simulink model "VCU_CS75_9_30"  (R2014a)
settings: Solver=FixedStepDiscrete  StartTime=0.0  StopTime=25  FixedStep=0.0005  RelTol=1e-3
undefined symbols (not defined in the file or in its folder): APAStatus_2D4, ecucoder_acal, I_SW01_L, LDW, ST_comd, TX2D4
libraries: simulink x881, ec5744lib x37
(part 28 of 30)

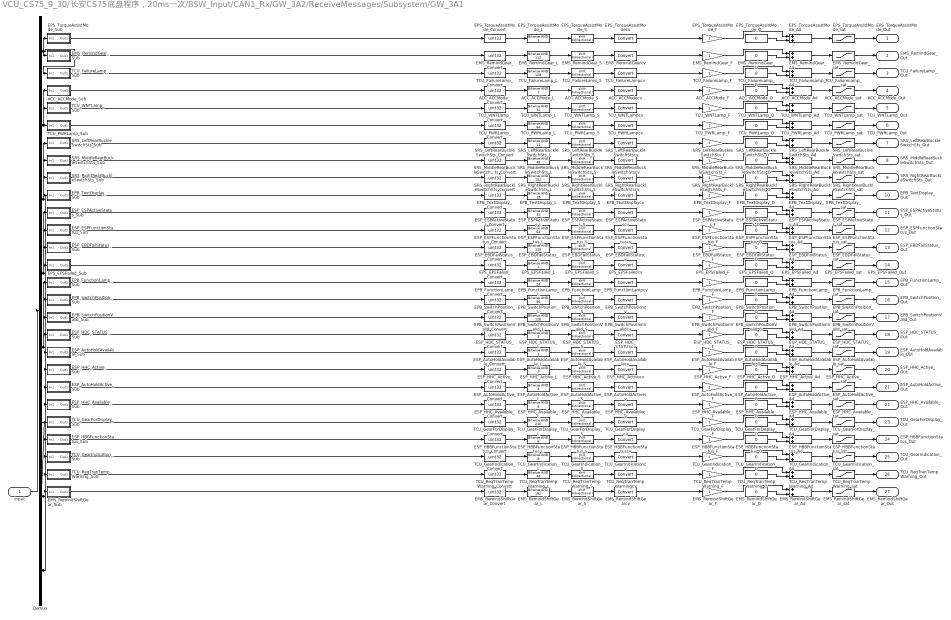
== system VCU_CS75_9_30/长安CS75底盘程序，20ms一次/BSW_Input/CAN1_Rx/GW_3A2/ReceiveMessages/Subsystem/GW_3A1 ==
  input : Inport
  ACC_ACCMode_Ad : Sum
  ACC_ACCMode_Convert : DataTypeConversion  OutDataTypeStr=uint32
  ACC_ACCMode_F : Gain
  ACC_ACCMode_L : simulink/Logic and Bit Operations/Bitwise Operator  logicop=AND  UseBitMask=on  BitMask=7  BitMaskRealWorld=Stored Integer
  ACC_ACCMode_O : Constant  Value=0  OutDataTypeStr=single
  ACC_ACCMode_S : ArithShift
  ACC_ACCMode_Sub : Subsystem
  ACC_ACCMode_sat : Saturate  UpperLimit=7  LowerLimit=0
  ACC_ACCModecv : DataTypeConversion
  Demux : Demux  Outputs=8
  EMS_RemindGear_Ad : Sum
  EMS_RemindGear_Convert : DataTypeConversion  OutDataTypeStr=uint32
  EMS_RemindGear_F : Gain
  EMS_RemindGear_L : simulink/Logic and Bit Operations/Bitwise Operator  logicop=AND  UseBitMask=on  BitMask=112  BitMaskRealWorld=Stored Integer
  EMS_RemindGear_O : Constant  Value=0  OutDataTypeStr=single
  EMS_RemindGear_S : ArithShift  BitShiftNumber=4
  EMS_RemindGear_Sub : Subsystem
  EMS_RemindGear_sat : Saturate  UpperLimit=7  LowerLimit=0
  EMS_RemindGearcv : DataTypeConversion
  EMS_RemindShiftGear_Ad : Sum
  EMS_RemindShiftGear_Convert : DataTypeConversion  OutDataTypeStr=uint32
  EMS_RemindShiftGear_F : Gain
  EMS_RemindShiftGear_L : simulink/Logic and Bit Operations/Bitwise Operator  logicop=AND  UseBitMask=on  BitMask=192  BitMaskRealWorld=Stored Integer
  EMS_RemindShiftGear_O : Constant  Value=0  OutDataTypeStr=single
  EMS_RemindShiftGear_S : ArithShift  BitShiftNumber=6
  EMS_RemindShiftGear_Sub : Subsystem
  EMS_RemindShiftGear_sat : Saturate  UpperLimit=3  LowerLimit=0
  EMS_RemindShiftGearcv : DataTypeConversion
  EPB_FunctionLamp_Ad : Sum
  EPB_FunctionLamp_Convert : DataTypeConversion  OutDataTypeStr=uint32
  EPB_FunctionLamp_F : Gain
  EPB_FunctionLamp_L : simulink/Logic and Bit Operations/Bitwise Operator  logicop=AND  UseBitMask=on  BitMask=24  BitMaskRealWorld=Stored Integer
  EPB_FunctionLamp_O : Constant  Value=0  OutDataTypeStr=single
  EPB_FunctionLamp_S : ArithShift  BitShiftNumber=3
  EPB_FunctionLamp_Sub : Subsystem
  EPB_FunctionLamp_sat : Saturate  UpperLimit=3  LowerLimit=0
  EPB_FunctionLampcv : DataTypeConversion
  EPB_SwitchPositionValid_Ad : Sum
  EPB_SwitchPositionValid_Convert : DataTypeConversion  OutDataTypeStr=uint32
  EPB_SwitchPositionValid_F : Gain
  EPB_SwitchPositionValid_L : simulink/Logic and Bit Operations/Bitwise Operator  logicop=AND  UseBitMask=on  BitMask=128  BitMaskRealWorld=Stored Integer
  EPB_SwitchPositionValid_O : Constant  Value=0  OutDataTypeStr=single
  EPB_SwitchPositionValid_S : ArithShift  BitShiftNumber=7
  EPB_SwitchPositionValid_Sub : Subsystem
  EPB_SwitchPositionValid_sat : Saturate  UpperLimit=1  LowerLimit=0
  EPB_SwitchPositionValidcv : DataTypeConversion
  EPB_SwitchPosition_Ad : Sum
  EPB_SwitchPosition_Convert : DataTypeConversion  OutDataTypeStr=uint32
  EPB_SwitchPosition_F : Gain
  EPB_SwitchPosition_L : simulink/Logic and Bit Operations/Bitwise Operator  logicop=AND  UseBitMask=on  BitMask=96  BitMaskRealWorld=Stored Integer
  EPB_SwitchPosition_O : Constant  Value=0  OutDataTypeStr=single
  EPB_SwitchPosition_S : ArithShift  BitShiftNumber=5
  EPB_SwitchPosition_Sub : Subsystem
  EPB_SwitchPosition_sat : Saturate  UpperLimit=3  LowerLimit=0
  EPB_SwitchPositioncv : DataTypeConversion
  EPB_TextDisplay_Ad : Sum
  EPB_TextDisplay_Convert : DataTypeConversion  OutDataTypeStr=uint32
  EPB_TextDisplay_F : Gain
  EPB_TextDisplay_L : simulink/Logic and Bit Operations/Bitwise Operator  logicop=AND  UseBitMask=on  BitMask=15  BitMaskRealWorld=Stored Integer
  EPB_TextDisplay_O : Constant  Value=0  OutDataTypeStr=single
  EPB_TextDisplay_S : ArithShift
  EPB_TextDisplay_Sub : Subsystem
  EPB_TextDisplay_sat : Saturate  UpperLimit=15  LowerLimit=0
  EPB_TextDisplaycv : DataTypeConversion
  EPS_EPSFailed_Ad : Sum
  EPS_EPSFailed_Convert : DataTypeConversion  OutDataTypeStr=uint32
  EPS_EPSFailed_F : Gain
  EPS_EPSFailed_L : simulink/Logic and Bit Operations/Bitwise Operator  logicop=AND  UseBitMask=on  BitMask=2  BitMaskRealWorld=Stored Integer
  EPS_EPSFailed_O : Constant  Value=0  OutDataTypeStr=single
  EPS_EPSFailed_S : ArithShift  BitShiftNumber=1
  EPS_EPSFailed_Sub : Subsystem
  EPS_EPSFailed_sat : Saturate  UpperLimit=1  LowerLimit=0
  EPS_EPSFailedcv : DataTypeConversion
  EPS_TorqueAssistMode_Ad : Sum
  EPS_TorqueAssistMode_Convert : DataTypeConversion  OutDataTypeStr=uint32
  EPS_TorqueAssistMode_F : Gain
  EPS_TorqueAssistMode_L : simulink/Logic and Bit Operations/Bitwise Operator  logicop=AND  UseBitMask=on  BitMask=3  BitMaskRealWorld=Stored Integer
  EPS_TorqueAssistMode_O : Constant  Value=0  OutDataTypeStr=single
  EPS_TorqueAssistMode_S : ArithShift
  EPS_TorqueAssistMode_Sub : Subsystem
  EPS_TorqueAssistMode_sat : Saturate  UpperLimit=3  LowerLimit=0
  EPS_TorqueAssistModecv : DataTypeConversion
  ESP_AutoHoldActive_Ad : Sum
  ESP_AutoHoldActive_Convert : DataTypeConversion  OutDataTypeStr=uint32
  ESP_AutoHoldActive_F : Gain
  ESP_AutoHoldActive_L : simulink/Logic and Bit Operations/Bitwise Operator  logicop=AND  UseBitMask=on  BitMask=4  BitMaskRealWorld=Stored Integer
  ESP_AutoHoldActive_O : Constant  Value=0  OutDataTypeStr=single
  ESP_AutoHoldActive_S : ArithShift  BitShiftNumber=2
  ESP_AutoHoldActive_Sub : Subsystem
  ESP_AutoHoldActive_sat : Saturate  UpperLimit=1  LowerLimit=0
  ESP_AutoHoldActivecv : DataTypeConversion
  ESP_AutoHoldAvailable_Ad : Sum
  ESP_AutoHoldAvailable_Convert : DataTypeConversion  OutDataTypeStr=uint32
  ESP_AutoHoldAvailable_F : Gain
  ESP_AutoHoldAvailable_L : simulink/Logic and Bit Operations/Bitwise Operator  logicop=AND  UseBitMask=on  BitMask=1  BitMaskRealWorld=Stored Integer
  ESP_AutoHoldAvailable_O : Constant  Value=0  OutDataTypeStr=single
  ESP_AutoHoldAvailable_S : ArithShift
  ESP_AutoHoldAvailable_Sub : Subsystem
  ESP_AutoHoldAvailable_sat : Saturate  UpperLimit=1  LowerLimit=0
  ESP_AutoHoldAvailablecv : DataTypeConversion
  ESP_EBDFailStatus_Ad : Sum
  ESP_EBDFailStatus_Convert : DataTypeConversion  OutDataTypeStr=uint32
  ESP_EBDFailStatus_F : Gain
  ESP_EBDFailStatus_L : simulink/Logic and Bit Operations/Bitwise Operator  logicop=AND  UseBitMask=on  BitMask=128  BitMaskRealWorld=Stored Integer
  ESP_EBDFailStatus_O : Constant  Value=0  OutDataTypeStr=single
  ESP_EBDFailStatus_S : ArithShift  BitShiftNumber=7
  ESP_EBDFailStatus_Sub : Subsystem
  ESP_EBDFailStatus_sat : Saturate  UpperLimit=1  LowerLimit=0
  ESP_EBDFailStatuscv : DataTypeConversion
  ESP_ESPActiveStatus_Ad : Sum
  ESP_ESPActiveStatus_Convert : DataTypeConversion  OutDataTypeStr=uint32
  ESP_ESPActiveStatus_F : Gain
  ESP_ESPActiveStatus_L : simulink/Logic and Bit Operations/Bitwise Operator  logicop=AND  UseBitMask=on  BitMask=32  BitMaskRealWorld=Stored Integer
  ESP_ESPActiveStatus_O : Constant  Value=0  OutDataTypeStr=single
  ESP_ESPActiveStatus_S : ArithShift  BitShiftNumber=5
  ESP_ESPActiveStatus_Sub : Subsystem
  ESP_ESPActiveStatus_sat : Saturate  UpperLimit=1  LowerLimit=0
  ESP_ESPActiveStatuscv : DataTypeConversion
  ESP_ESPFunctionStatus_Ad : Sum
  ESP_ESPFunctionStatus_Convert : DataTypeConversion  OutDataTypeStr=uint32
  ESP_ESPFunctionStatus_F : Gain
  ESP_ESPFunctionStatus_L : simulink/Logic and Bit Operations/Bitwise Operator  logicop=AND  UseBitMask=on  BitMask=64  BitMaskRealWorld=Stored Integer
  ESP_ESPFunctionStatus_O : Constant  Value=0  OutDataTypeStr=single
  ESP_ESPFunctionStatus_S : ArithShift  BitShiftNumber=6
  ESP_ESPFunctionStatus_Sub : Subsystem
  ESP_ESPFunctionStatus_sat : Saturate  UpperLimit=1  LowerLimit=0
  ESP_ESPFunctionStatuscv : DataTypeConversion
  ESP_HBBFunctionStatus_Ad : Sum
  ESP_HBBFunctionStatus_Convert : DataTypeConversion  OutDataTypeStr=uint32
  ESP_HBBFunctionStatus_F : Gain
  ESP_HBBFunctionStatus_L : simulink/Logic and Bit Operations/Bitwise Operator  logicop=AND  UseBitMask=on  BitMask=6  BitMaskRealWorld=Stored Integer
  ESP_HBBFunctionStatus_O : Constant  Value=0  OutDataTypeStr=single
  ESP_HBBFunctionStatus_S : ArithShift  BitShiftNumber=1
  ESP_HBBFunctionStatus_Sub : Subsystem
  ESP_HBBFunctionStatus_sat : Saturate  UpperLimit=3  LowerLimit=0
  ESP_HBBFunctionStatuscv : DataTypeConversion
  ESP_HDC_STATUS_Ad : Sum
  ESP_HDC_STATUS_Convert : DataTypeConversion  OutDataTypeStr=uint32
  ESP_HDC_STATUS_F : Gain
  ESP_HDC_STATUS_L : simulink/Logic and Bit Operations/Bitwise Operator  logicop=AND  UseBitMask=on  BitMask=3  BitMaskRealWorld=Stored Integer
  ESP_HDC_STATUS_O : Constant  Value=0  OutDataTypeStr=single
  ESP_HDC_STATUS_S : ArithShift
  ESP_HDC_STATUS_Sub : Subsystem
  ESP_HDC_STATUS_sat : Saturate  UpperLimit=3  LowerLimit=0
  ESP_HDC_STATUScv : DataTypeConversion
  ESP_HHC_Active_Ad : Sum
  ESP_HHC_Active_Convert : DataTypeConversion  OutDataTypeStr=uint32
  ESP_HHC_Active_F : Gain
  ESP_HHC_Active_L : simulink/Logic and Bit Operations/Bitwise Operator  logicop=AND  UseBitMask=on  BitMask=2  BitMaskRealWorld=Stored Integer
  ESP_HHC_Active_O : Constant  Value=0  OutDataTypeStr=single
  ESP_HHC_Active_S : ArithShift  BitShiftNumber=1
  ESP_HHC_Active_Sub : Subsystem
  ESP_HHC_Active_sat : Saturate  UpperLimit=1  LowerLimit=0
  ESP_HHC_Activecv : DataTypeConversion
  ESP_HHC_Available_Ad : Sum
  ESP_HHC_Available_Convert : DataTypeConversion  OutDataTypeStr=uint32
  ESP_HHC_Available_F : Gain
  ESP_HHC_Available_L : simulink/Logic and Bit Operations/Bitwise Operator  logicop=AND  UseBitMask=on  BitMask=8  BitMaskRealWorld=Stored Integer
  ESP_HHC_Available_O : Constant  Value=0  OutDataTypeStr=single
  ESP_HHC_Available_S : ArithShift  BitShiftNumber=3
  ESP_HHC_Available_Sub : Subsystem
  ESP_HHC_Available_sat : Saturate  UpperLimit=1  LowerLimit=0
  ESP_HHC_Availablecv : DataTypeConversion
  SRS_LeftRearBuckleSwitchSts_Ad : Sum
  SRS_LeftRearBuckleSwitchSts_Convert : DataTypeConversion  OutDataTypeStr=uint32
  SRS_LeftRearBuckleSwitchSts_F : Gain
  SRS_LeftRearBuckleSwitchSts_L : simulink/Logic and Bit Operations/Bitwise Operator  logicop=AND  UseBitMask=on  BitMask=12  BitMaskRealWorld=Stored Integer
  SRS_LeftRearBuckleSwitchSts_O : Constant  Value=0  OutDataTypeStr=single
  SRS_LeftRearBuckleSwitchSts_S : ArithShift  BitShiftNumber=2
  SRS_LeftRearBuckleSwitchSts_Sub : Subsystem
  SRS_LeftRearBuckleSwitchSts_sat : Saturate  UpperLimit=3  LowerLimit=0
  SRS_LeftRearBuckleSwitchStscv : DataTypeConversion
  SRS_MiddleRearBuckleSwitchSts_Ad : Sum
  SRS_MiddleRearBuckleSwitchSts_Convert : DataTypeConversion  OutDataTypeStr=uint32
  SRS_MiddleRearBuckleSwitchSts_F : Gain
  SRS_MiddleRearBuckleSwitchSts_L : simulink/Logic and Bit Operations/Bitwise Operator  logicop=AND  UseBitMask=on  BitMask=48  BitMaskRealWorld=Stored Integer
  SRS_MiddleRearBuckleSwitchSts_O : Constant  Value=0  OutDataTypeStr=single
  SRS_MiddleRearBuckleSwitchSts_S : ArithShift  BitShiftNumber=4
  SRS_MiddleRearBuckleSwitchSts_Sub : Subsystem
  SRS_MiddleRearBuckleSwitchSts_sat : Saturate  UpperLimit=3  LowerLimit=0
  SRS_MiddleRearBuckleSwitchStscv : DataTypeConversion
  SRS_RightRearBuckleSwitchSts_Ad : Sum
  SRS_RightRearBuckleSwitchSts_Convert : DataTypeConversion  OutDataTypeStr=uint32
  SRS_RightRearBuckleSwitchSts_F : Gain
  SRS_RightRearBuckleSwitchSts_L : simulink/Logic and Bit Operations/Bitwise Operator  logicop=AND  UseBitMask=on  BitMask=192  BitMaskRealWorld=Stored Integer
  SRS_RightRearBuckleSwitchSts_O : Constant  Value=0  OutDataTypeStr=single
  SRS_RightRearBuckleSwitchSts_S : ArithShift  BitShiftNumber=6
  SRS_RightRearBuckleSwitchSts_Sub : Subsystem
  SRS_RightRearBuckleSwitchSts_sat : Saturate  UpperLimit=3  LowerLimit=0
  SRS_RightRearBuckleSwitchStscv : DataTypeConversion
  TCU_FailureLamp_Ad : Sum
  TCU_FailureLamp_Convert : DataTypeConversion  OutDataTypeStr=uint32
  TCU_FailureLamp_F : Gain
  TCU_FailureLamp_L : simulink/Logic and Bit Operations/Bitwise Operator  logicop=AND  UseBitMask=on  BitMask=128  BitMaskRealWorld=Stored Integer
  TCU_FailureLamp_O : Constant  Value=0  OutDataTypeStr=single
  TCU_FailureLamp_S : ArithShift  BitShiftNumber=7
  TCU_FailureLamp_Sub : Subsystem
  TCU_FailureLamp_sat : Saturate  UpperLimit=1  LowerLimit=0
  TCU_FailureLampcv : DataTypeConversion
  TCU_GearForDisplay_Ad : Sum
  TCU_GearForDisplay_Convert : DataTypeConversion  OutDataTypeStr=uint32
  TCU_GearForDisplay_F : Gain
  TCU_GearForDisplay_L : simulink/Logic and Bit Operations/Bitwise Operator  logicop=AND  UseBitMask=on  BitMask=240  BitMaskRealWorld=Stored Integer
  TCU_GearForDisplay_O : Constant  Value=0  OutDataTypeStr=single
  TCU_GearForDisplay_S : ArithShift  BitShiftNumber=4
  TCU_GearForDisplay_Sub : Subsystem
  TCU_GearForDisplay_sat : Saturate  UpperLimit=15  LowerLimit=0
  TCU_GearForDisplaycv : DataTypeConversion
  TCU_GearIndication_Ad : Sum
  TCU_GearIndication_Convert : DataTypeConversion  OutDataTypeStr=uint32
  TCU_GearIndication_F : Gain
  TCU_GearIndication_L : simulink/Logic and Bit Operations/Bitwise Operator  logicop=AND  UseBitMask=on  BitMask=8  BitMaskRealWorld=Stored Integer
  TCU_GearIndication_O : Constant  Value=0  OutDataTypeStr=single
  TCU_GearIndication_S : ArithShift  BitShiftNumber=3
  TCU_GearIndication_Sub : Subsystem
  TCU_GearIndication_sat : Saturate  UpperLimit=1  LowerLimit=0
  TCU_GearIndicationcv : DataTypeConversion
  TCU_PWRLamp_Ad : Sum
  TCU_PWRLamp_Convert : DataTypeConversion  OutDataTypeStr=uint32
  TCU_PWRLamp_F : Gain
  TCU_PWRLamp_L : simulink/Logic and Bit Operations/Bitwise Operator  logicop=AND  UseBitMask=on  BitMask=64  BitMaskRealWorld=Stored Integer
  TCU_PWRLamp_O : Constant  Value=0  OutDataTypeStr=single
  TCU_PWRLamp_S : ArithShift  BitShiftNumber=6
  TCU_PWRLamp_Sub : Subsystem
  TCU_PWRLamp_sat : Saturate  UpperLimit=1  LowerLimit=0
  TCU_PWRLampcv : DataTypeConversion
  TCU_ReqTranTempWarning_Ad : Sum
  TCU_ReqTranTempWarning_Convert : DataTypeConversion  OutDataTypeStr=uint32
  TCU_ReqTranTempWarning_F : Gain
  TCU_ReqTranTempWarning_L : simulink/Logic and Bit Operations/Bitwise Operator  logicop=AND  UseBitMask=on  BitMask=48  BitMaskRealWorld=Stored Integer
  TCU_ReqTranTempWarning_O : Constant  Value=0  OutDataTypeStr=single
  TCU_ReqTranTempWarning_S : ArithShift  BitShiftNumber=4
  TCU_ReqTranTempWarning_Sub : Subsystem
  TCU_ReqTranTempWarning_sat : Saturate  UpperLimit=3  LowerLimit=0
  TCU_ReqTranTempWarningcv : DataTypeConversion
  TCU_WNTLamp_Ad : Sum
  TCU_WNTLamp_Convert : DataTypeConversion  OutDataTypeStr=uint32
  TCU_WNTLamp_F : Gain
  TCU_WNTLamp_L : simulink/Logic and Bit Operations/Bitwise Operator  logicop=AND  UseBitMask=on  BitMask=32  BitMaskRealWorld=Stored Integer
  TCU_WNTLamp_O : Constant  Value=0  OutDataTypeStr=single
  TCU_WNTLamp_S : ArithShift  BitShiftNumber=5
  TCU_WNTLamp_Sub : Subsystem
  TCU_WNTLamp_sat : Saturate  UpperLimit=1  LowerLimit=0
  TCU_WNTLampcv : DataTypeConversion
  EPS_TorqueAssistMode_Out : Outport
  EMS_RemindGear_Out : Outport  Port=2
  TCU_FailureLamp_Out : Outport  Port=3
  ACC_ACCMode_Out : Outport  Port=4
  TCU_WNTLamp_Out : Outport  Port=5
  TCU_PWRLamp_Out : Outport  Port=6
  SRS_LeftRearBuckleSwitchSts_Out : Outport  Port=7
  SRS_MiddleRearBuckleSwitchSts_Out : Outport  Port=8
  SRS_RightRearBuckleSwitchSts_Out : Outport  Port=9
  EPB_TextDisplay_Out : Outport  Port=10
  ESP_ESPActiveStatus_Out : Outport  Port=11
  ESP_ESPFunctionStatus_Out : Outport  Port=12
  ESP_EBDFailStatus_Out : Outport  Port=13
  EPS_EPSFailed_Out : Outport  Port=14
  EPB_FunctionLamp_Out : Outport  Port=15
  EPB_SwitchPosition_Out : Outport  Port=16
  EPB_SwitchPositionValid_Out : Outport  Port=17
  ESP_HDC_STATUS_Out : Outport  Port=18
  ESP_AutoHoldAvailable_Out : Outport  Port=19
  ESP_HHC_Active_Out : Outport  Port=20
  ESP_AutoHoldActive_Out : Outport  Port=21
  ESP_HHC_Available_Out : Outport  Port=22
  TCU_GearForDisplay_Out : Outport  Port=23
  ESP_HBBFunctionStatus_Out : Outport  Port=24
  TCU_GearIndication_Out : Outport  Port=25
  TCU_ReqTranTempWarning_Out : Outport  Port=26
  EMS_RemindShiftGear_Out : Outport  Port=27
  wires:
  input/1 -> Demux/1
  EMS_RemindShiftGearcv/1 -> EMS_RemindShiftGear_F/1
  EMS_RemindShiftGear_S/1 -> EMS_RemindShiftGearcv/1
  EMS_RemindShiftGear_L/1 -> EMS_RemindShiftGear_S/1
  EMS_RemindShiftGear_Convert/1 -> EMS_RemindShiftGear_L/1
  EMS_RemindShiftGear_Sub/1(Out1) -> EMS_RemindShiftGear_Convert/1
  EMS_RemindShiftGear_sat/1 -> EMS_RemindShiftGear_Out/1
  EMS_RemindShiftGear_Ad/1 -> EMS_RemindShiftGear_sat/1
  EMS_RemindShiftGear_O/1 -> EMS_RemindShiftGear_Ad/2
  EMS_RemindShiftGear_F/1 -> EMS_RemindShiftGear_Ad/1
  TCU_ReqTranTempWarningcv/1 -> TCU_ReqTranTempWarning_F/1
  TCU_ReqTranTempWarning_S/1 -> TCU_ReqTranTempWarningcv/1
  TCU_ReqTranTempWarning_L/1 -> TCU_ReqTranTempWarning_S/1
  TCU_ReqTranTempWarning_Convert/1 -> TCU_ReqTranTempWarning_L/1
  TCU_ReqTranTempWarning_Sub/1(Out1) -> TCU_ReqTranTempWarning_Convert/1
  TCU_ReqTranTempWarning_sat/1 -> TCU_ReqTranTempWarning_Out/1
  TCU_ReqTranTempWarning_Ad/1 -> TCU_ReqTranTempWarning_sat/1
  TCU_ReqTranTempWarning_O/1 -> TCU_ReqTranTempWarning_Ad/2
  TCU_ReqTranTempWarning_F/1 -> TCU_ReqTranTempWarning_Ad/1
  TCU_GearIndicationcv/1 -> TCU_GearIndication_F/1
  TCU_GearIndication_S/1 -> TCU_GearIndicationcv/1
  TCU_GearIndication_L/1 -> TCU_GearIndication_S/1
  TCU_GearIndication_Convert/1 -> TCU_GearIndication_L/1
  TCU_GearIndication_Sub/1(Out1) -> TCU_GearIndication_Convert/1
  TCU_GearIndication_sat/1 -> TCU_GearIndication_Out/1
  TCU_GearIndication_Ad/1 -> TCU_GearIndication_sat/1
  TCU_GearIndication_O/1 -> TCU_GearIndication_Ad/2
  TCU_GearIndication_F/1 -> TCU_GearIndication_Ad/1
  ESP_HBBFunctionStatuscv/1 -> ESP_HBBFunctionStatus_F/1
  ESP_HBBFunctionStatus_S/1 -> ESP_HBBFunctionStatuscv/1
  ESP_HBBFunctionStatus_L/1 -> ESP_HBBFunctionStatus_S/1
  ESP_HBBFunctionStatus_Convert/1 -> ESP_HBBFunctionStatus_L/1
  ESP_HBBFunctionStatus_Sub/1(Out1) -> ESP_HBBFunctionStatus_Convert/1
  Demux/8 -> EMS_RemindShiftGear_Sub/1(In1), TCU_ReqTranTempWarning_Sub/1(In1), TCU_GearIndication_Sub/1(In1), ESP_HBBFunctionStatus_Sub/1(In1)
  ESP_HBBFunctionStatus_sat/1 -> ESP_HBBFunctionStatus_Out/1
  ESP_HBBFunctionStatus_Ad/1 -> ESP_HBBFunctionStatus_sat/1
  ESP_HBBFunctionStatus_O/1 -> ESP_HBBFunctionStatus_Ad/2
  ESP_HBBFunctionStatus_F/1 -> ESP_HBBFunctionStatus_Ad/1
  TCU_GearForDisplaycv/1 -> TCU_GearForDisplay_F/1
  TCU_GearForDisplay_S/1 -> TCU_GearForDisplaycv/1
  TCU_GearForDisplay_L/1 -> TCU_GearForDisplay_S/1
  TCU_GearForDisplay_Convert/1 -> TCU_GearForDisplay_L/1
  TCU_GearForDisplay_Sub/1(Out1) -> TCU_GearForDisplay_Convert/1
  TCU_GearForDisplay_sat/1 -> TCU_GearForDisplay_Out/1
  TCU_GearForDisplay_Ad/1 -> TCU_GearForDisplay_sat/1
  TCU_GearForDisplay_O/1 -> TCU_GearForDisplay_Ad/2
  TCU_GearForDisplay_F/1 -> TCU_GearForDisplay_Ad/1
  ESP_HHC_Availablecv/1 -> ESP_HHC_Available_F/1
  ESP_HHC_Available_S/1 -> ESP_HHC_Availablecv/1
  ESP_HHC_Available_L/1 -> ESP_HHC_Available_S/1
  ESP_HHC_Available_Convert/1 -> ESP_HHC_Available_L/1
  ESP_HHC_Available_Sub/1(Out1) -> ESP_HHC_Available_Convert/1
  ESP_HHC_Available_sat/1 -> ESP_HHC_Available_Out/1
  ESP_HHC_Available_Ad/1 -> ESP_HHC_Available_sat/1
  ESP_HHC_Available_O/1 -> ESP_HHC_Available_Ad/2
  ESP_HHC_Available_F/1 -> ESP_HHC_Available_Ad/1
  ESP_AutoHoldActivecv/1 -> ESP_AutoHoldActive_F/1
  ESP_AutoHoldActive_S/1 -> ESP_AutoHoldActivecv/1
  ESP_AutoHoldActive_L/1 -> ESP_AutoHoldActive_S/1
  ESP_AutoHoldActive_Convert/1 -> ESP_AutoHoldActive_L/1
  ESP_AutoHoldActive_Sub/1(Out1) -> ESP_AutoHoldActive_Convert/1
  ESP_AutoHoldActive_sat/1 -> ESP_AutoHoldActive_Out/1
  ESP_AutoHoldActive_Ad/1 -> ESP_AutoHoldActive_sat/1
  ESP_AutoHoldActive_O/1 -> ESP_AutoHoldActive_Ad/2
  ESP_AutoHoldActive_F/1 -> ESP_AutoHoldActive_Ad/1
  ESP_HHC_Activecv/1 -> ESP_HHC_Active_F/1
  ESP_HHC_Active_S/1 -> ESP_HHC_Activecv/1
  ESP_HHC_Active_L/1 -> ESP_HHC_Active_S/1
  ESP_HHC_Active_Convert/1 -> ESP_HHC_Active_L/1
  ESP_HHC_Active_Sub/1(Out1) -> ESP_HHC_Active_Convert/1
  ESP_HHC_Active_sat/1 -> ESP_HHC_Active_Out/1
  ESP_HHC_Active_Ad/1 -> ESP_HHC_Active_sat/1
  ESP_HHC_Active_O/1 -> ESP_HHC_Active_Ad/2
  ESP_HHC_Active_F/1 -> ESP_HHC_Active_Ad/1
  ESP_AutoHoldAvailablecv/1 -> ESP_AutoHoldAvailable_F/1
  ESP_AutoHoldAvailable_S/1 -> ESP_AutoHoldAvailablecv/1
  ESP_AutoHoldAvailable_L/1 -> ESP_AutoHoldAvailable_S/1
  ESP_AutoHoldAvailable_Convert/1 -> ESP_AutoHoldAvailable_L/1
  ESP_AutoHoldAvailable_Sub/1(Out1) -> ESP_AutoHoldAvailable_Convert/1
  Demux/7 -> TCU_GearForDisplay_Sub/1(In1), ESP_HHC_Available_Sub/1(In1), ESP_AutoHoldActive_Sub/1(In1), ESP_HHC_Active_Sub/1(In1), ESP_AutoHoldAvailable_Sub/1(In1)
  ESP_AutoHoldAvailable_sat/1 -> ESP_AutoHoldAvailable_Out/1
  ESP_AutoHoldAvailable_Ad/1 -> ESP_AutoHoldAvailable_sat/1
  ESP_AutoHoldAvailable_O/1 -> ESP_AutoHoldAvailable_Ad/2
  ESP_AutoHoldAvailable_F/1 -> ESP_AutoHoldAvailable_Ad/1
  ESP_HDC_STATUScv/1 -> ESP_HDC_STATUS_F/1
  ESP_HDC_STATUS_S/1 -> ESP_HDC_STATUScv/1
  ESP_HDC_STATUS_L/1 -> ESP_HDC_STATUS_S/1
  ESP_HDC_STATUS_Convert/1 -> ESP_HDC_STATUS_L/1
  ESP_HDC_STATUS_Sub/1(Out1) -> ESP_HDC_STATUS_Convert/1
  Demux/6 -> ESP_HDC_STATUS_Sub/1(In1)
  ESP_HDC_STATUS_sat/1 -> ESP_HDC_STATUS_Out/1
  ESP_HDC_STATUS_Ad/1 -> ESP_HDC_STATUS_sat/1
  ESP_HDC_STATUS_O/1 -> ESP_HDC_STATUS_Ad/2
  ESP_HDC_STATUS_F/1 -> ESP_HDC_STATUS_Ad/1
  EPB_SwitchPositionValidcv/1 -> EPB_SwitchPositionValid_F/1
  EPB_SwitchPositionValid_S/1 -> EPB_SwitchPositionValidcv/1
  EPB_SwitchPositionValid_L/1 -> EPB_SwitchPositionValid_S/1
  EPB_SwitchPositionValid_Convert/1 -> EPB_SwitchPositionValid_L/1
  EPB_SwitchPositionValid_Sub/1(Out1) -> EPB_SwitchPositionValid_Convert/1
  EPB_SwitchPositionValid_sat/1 -> EPB_SwitchPositionValid_Out/1
  EPB_SwitchPositionValid_Ad/1 -> EPB_SwitchPositionValid_sat/1
  EPB_SwitchPositionValid_O/1 -> EPB_SwitchPositionValid_Ad/2
  EPB_SwitchPositionValid_F/1 -> EPB_SwitchPositionValid_Ad/1
  EPB_SwitchPositioncv/1 -> EPB_SwitchPosition_F/1
  EPB_SwitchPosition_S/1 -> EPB_SwitchPositioncv/1
  EPB_SwitchPosition_L/1 -> EPB_SwitchPosition_S/1
  EPB_SwitchPosition_Convert/1 -> EPB_SwitchPosition_L/1
  EPB_SwitchPosition_Sub/1(Out1) -> EPB_SwitchPosition_Convert/1
  EPB_SwitchPosition_sat/1 -> EPB_SwitchPosition_Out/1
  EPB_SwitchPosition_Ad/1 -> EPB_SwitchPosition_sat/1
  EPB_SwitchPosition_O/1 -> EPB_SwitchPosition_Ad/2
  EPB_SwitchPosition_F/1 -> EPB_SwitchPosition_Ad/1
  EPB_FunctionLampcv/1 -> EPB_FunctionLamp_F/1
  EPB_FunctionLamp_S/1 -> EPB_FunctionLampcv/1
  EPB_FunctionLamp_L/1 -> EPB_FunctionLamp_S/1
  EPB_FunctionLamp_Convert/1 -> EPB_FunctionLamp_L/1
  EPB_FunctionLamp_Sub/1(Out1) -> EPB_FunctionLamp_Convert/1
  EPB_FunctionLamp_sat/1 -> EPB_FunctionLamp_Out/1
  EPB_FunctionLamp_Ad/1 -> EPB_FunctionLamp_sat/1
  EPB_FunctionLamp_O/1 -> EPB_FunctionLamp_Ad/2
  EPB_FunctionLamp_F/1 -> EPB_FunctionLamp_Ad/1
  EPS_EPSFailedcv/1 -> EPS_EPSFailed_F/1
  EPS_EPSFailed_S/1 -> EPS_EPSFailedcv/1
  EPS_EPSFailed_L/1 -> EPS_EPSFailed_S/1
  EPS_EPSFailed_Convert/1 -> EPS_EPSFailed_L/1
  EPS_EPSFailed_Sub/1(Out1) -> EPS_EPSFailed_Convert/1
  Demux/5 -> EPB_SwitchPositionValid_Sub/1(In1), EPB_SwitchPosition_Sub/1(In1), EPB_FunctionLamp_Sub/1(In1), EPS_EPSFailed_Sub/1(In1)
  EPS_EPSFailed_sat/1 -> EPS_EPSFailed_Out/1
  EPS_EPSFailed_Ad/1 -> EPS_EPSFailed_sat/1
  EPS_EPSFailed_O/1 -> EPS_EPSFailed_Ad/2
  EPS_EPSFailed_F/1 -> EPS_EPSFailed_Ad/1
  ESP_EBDFailStatuscv/1 -> ESP_EBDFailStatus_F/1
  ESP_EBDFailStatus_S/1 -> ESP_EBDFailStatuscv/1
  ESP_EBDFailStatus_L/1 -> ESP_EBDFailStatus_S/1
  ESP_EBDFailStatus_Convert/1 -> ESP_EBDFailStatus_L/1
  ESP_EBDFailStatus_Sub/1(Out1) -> ESP_EBDFailStatus_Convert/1
  ESP_EBDFailStatus_sat/1 -> ESP_EBDFailStatus_Out/1
  ESP_EBDFailStatus_Ad/1 -> ESP_EBDFailStatus_sat/1
  ESP_EBDFailStatus_O/1 -> ESP_EBDFailStatus_Ad/2
  ESP_EBDFailStatus_F/1 -> ESP_EBDFailStatus_Ad/1
  ESP_ESPFunctionStatuscv/1 -> ESP_ESPFunctionStatus_F/1
  ESP_ESPFunctionStatus_S/1 -> ESP_ESPFunctionStatuscv/1
  ESP_ESPFunctionStatus_L/1 -> ESP_ESPFunctionStatus_S/1
  ESP_ESPFunctionStatus_Convert/1 -> ESP_ESPFunctionStatus_L/1
  ESP_ESPFunctionStatus_Sub/1(Out1) -> ESP_ESPFunctionStatus_Convert/1
  ESP_ESPFunctionStatus_sat/1 -> ESP_ESPFunctionStatus_Out/1
  ESP_ESPFunctionStatus_Ad/1 -> ESP_ESPFunctionStatus_sat/1
  ESP_ESPFunctionStatus_O/1 -> ESP_ESPFunctionStatus_Ad/2
  ESP_ESPFunctionStatus_F/1 -> ESP_ESPFunctionStatus_Ad/1
  ESP_ESPActiveStatuscv/1 -> ESP_ESPActiveStatus_F/1
  ESP_ESPActiveStatus_S/1 -> ESP_ESPActiveStatuscv/1
  ESP_ESPActiveStatus_L/1 -> ESP_ESPActiveStatus_S/1
  ESP_ESPActiveStatus_Convert/1 -> ESP_ESPActiveStatus_L/1
  ESP_ESPActiveStatus_Sub/1(Out1) -> ESP_ESPActiveStatus_Convert/1
  ESP_ESPActiveStatus_sat/1 -> ESP_ESPActiveStatus_Out/1
  ESP_ESPActiveStatus_Ad/1 -> ESP_ESPActiveStatus_sat/1
  ESP_ESPActiveStatus_O/1 -> ESP_ESPActiveStatus_Ad/2
  ESP_ESPActiveStatus_F/1 -> ESP_ESPActiveStatus_Ad/1
  EPB_TextDisplaycv/1 -> EPB_TextDisplay_F/1
  EPB_TextDisplay_S/1 -> EPB_TextDisplaycv/1
  EPB_TextDisplay_L/1 -> EPB_TextDisplay_S/1
  EPB_TextDisplay_Convert/1 -> EPB_TextDisplay_L/1
  EPB_TextDisplay_Sub/1(Out1) -> EPB_TextDisplay_Convert/1
  Demux/4 -> ESP_EBDFailStatus_Sub/1(In1), ESP_ESPFunctionStatus_Sub/1(In1), ESP_ESPActiveStatus_Sub/1(In1), EPB_TextDisplay_Sub/1(In1)
  EPB_TextDisplay_sat/1 -> EPB_TextDisplay_Out/1
  EPB_TextDisplay_Ad/1 -> EPB_TextDisplay_sat/1
  EPB_TextDisplay_O/1 -> EPB_TextDisplay_Ad/2
  EPB_TextDisplay_F/1 -> EPB_TextDisplay_Ad/1
  SRS_RightRearBuckleSwitchStscv/1 -> SRS_RightRearBuckleSwitchSts_F/1
  SRS_RightRearBuckleSwitchSts_S/1 -> SRS_RightRearBuckleSwitchStscv/1
  SRS_RightRearBuckleSwitchSts_L/1 -> SRS_RightRearBuckleSwitchSts_S/1
  SRS_RightRearBuckleSwitchSts_Convert/1 -> SRS_RightRearBuckleSwitchSts_L/1
  SRS_RightRearBuckleSwitchSts_Sub/1(Out1) -> SRS_RightRearBuckleSwitchSts_Convert/1
  SRS_RightRearBuckleSwitchSts_sat/1 -> SRS_RightRearBuckleSwitchSts_Out/1
  SRS_RightRearBuckleSwitchSts_Ad/1 -> SRS_RightRearBuckleSwitchSts_sat/1
  SRS_RightRearBuckleSwitchSts_O/1 -> SRS_RightRearBuckleSwitchSts_Ad/2
  SRS_RightRearBuckleSwitchSts_F/1 -> SRS_RightRearBuckleSwitchSts_Ad/1
  SRS_MiddleRearBuckleSwitchStscv/1 -> SRS_MiddleRearBuckleSwitchSts_F/1
  SRS_MiddleRearBuckleSwitchSts_S/1 -> SRS_MiddleRearBuckleSwitchStscv/1
  SRS_MiddleRearBuckleSwitchSts_L/1 -> SRS_MiddleRearBuckleSwitchSts_S/1
  SRS_MiddleRearBuckleSwitchSts_Convert/1 -> SRS_MiddleRearBuckleSwitchSts_L/1
  SRS_MiddleRearBuckleSwitchSts_Sub/1(Out1) -> SRS_MiddleRearBuckleSwitchSts_Convert/1
  SRS_MiddleRearBuckleSwitchSts_sat/1 -> SRS_MiddleRearBuckleSwitchSts_Out/1
  SRS_MiddleRearBuckleSwitchSts_Ad/1 -> SRS_MiddleRearBuckleSwitchSts_sat/1
  SRS_MiddleRearBuckleSwitchSts_O/1 -> SRS_MiddleRearBuckleSwitchSts_Ad/2
  SRS_MiddleRearBuckleSwitchSts_F/1 -> SRS_MiddleRearBuckleSwitchSts_Ad/1
  SRS_LeftRearBuckleSwitchStscv/1 -> SRS_LeftRearBuckleSwitchSts_F/1
  SRS_LeftRearBuckleSwitchSts_S/1 -> SRS_LeftRearBuckleSwitchStscv/1
  SRS_LeftRearBuckleSwitchSts_L/1 -> SRS_LeftRearBuckleSwitchSts_S/1
  SRS_LeftRearBuckleSwitchSts_Convert/1 -> SRS_LeftRearBuckleSwitchSts_L/1
  SRS_LeftRearBuckleSwitchSts_Sub/1(Out1) -> SRS_LeftRearBuckleSwitchSts_Convert/1
  Demux/3 -> SRS_RightRearBuckleSwitchSts_Sub/1(In1), SRS_MiddleRearBuckleSwitchSts_Sub/1(In1), SRS_LeftRearBuckleSwitchSts_Sub/1(In1)
  SRS_LeftRearBuckleSwitchSts_sat/1 -> SRS_LeftRearBuckleSwitchSts_Out/1
  SRS_LeftRearBuckleSwitchSts_Ad/1 -> SRS_LeftRearBuckleSwitchSts_sat/1
  SRS_LeftRearBuckleSwitchSts_O/1 -> SRS_LeftRearBuckleSwitchSts_Ad/2
  SRS_LeftRearBuckleSwitchSts_F/1 -> SRS_LeftRearBuckleSwitchSts_Ad/1
  TCU_PWRLampcv/1 -> TCU_PWRLamp_F/1
  TCU_PWRLamp_S/1 -> TCU_PWRLampcv/1
  TCU_PWRLamp_L/1 -> TCU_PWRLamp_S/1
  TCU_PWRLamp_Convert/1 -> TCU_PWRLamp_L/1
  TCU_PWRLamp_Sub/1(Out1) -> TCU_PWRLamp_Convert/1
  TCU_PWRLamp_sat/1 -> TCU_PWRLamp_Out/1
  TCU_PWRLamp_Ad/1 -> TCU_PWRLamp_sat/1
  TCU_PWRLamp_O/1 -> TCU_PWRLamp_Ad/2
  TCU_PWRLamp_F/1 -> TCU_PWRLamp_Ad/1
  TCU_WNTLampcv/1 -> TCU_WNTLamp_F/1
  TCU_WNTLamp_S/1 -> TCU_WNTLampcv/1
  TCU_WNTLamp_L/1 -> TCU_WNTLamp_S/1
  TCU_WNTLamp_Convert/1 -> TCU_WNTLamp_L/1
  TCU_WNTLamp_Sub/1(Out1) -> TCU_WNTLamp_Convert/1
  TCU_WNTLamp_sat/1 -> TCU_WNTLamp_Out/1
  TCU_WNTLamp_Ad/1 -> TCU_WNTLamp_sat/1
  TCU_WNTLamp_O/1 -> TCU_WNTLamp_Ad/2
  TCU_WNTLamp_F/1 -> TCU_WNTLamp_Ad/1
  ACC_ACCModecv/1 -> ACC_ACCMode_F/1
  ACC_ACCMode_S/1 -> ACC_ACCModecv/1
  ACC_ACCMode_L/1 -> ACC_ACCMode_S/1
  ACC_ACCMode_Convert/1 -> ACC_ACCMode_L/1
  ACC_ACCMode_Sub/1(Out1) -> ACC_ACCMode_Convert/1
  Demux/2 -> TCU_PWRLamp_Sub/1(In1), TCU_WNTLamp_Sub/1(In1), ACC_ACCMode_Sub/1(In1)
  ACC_ACCMode_sat/1 -> ACC_ACCMode_Out/1
  ACC_ACCMode_Ad/1 -> ACC_ACCMode_sat/1
  ACC_ACCMode_O/1 -> ACC_ACCMode_Ad/2
  ACC_ACCMode_F/1 -> ACC_ACCMode_Ad/1
  TCU_FailureLampcv/1 -> TCU_FailureLamp_F/1
  TCU_FailureLamp_S/1 -> TCU_FailureLampcv/1
  TCU_FailureLamp_L/1 -> TCU_FailureLamp_S/1
  TCU_FailureLamp_Convert/1 -> TCU_FailureLamp_L/1
  TCU_FailureLamp_Sub/1(Out1) -> TCU_FailureLamp_Convert/1
  TCU_FailureLamp_sat/1 -> TCU_FailureLamp_Out/1
  TCU_FailureLamp_Ad/1 -> TCU_FailureLamp_sat/1
  TCU_FailureLamp_O/1 -> TCU_FailureLamp_Ad/2
  TCU_FailureLamp_F/1 -> TCU_FailureLamp_Ad/1
  EMS_RemindGearcv/1 -> EMS_RemindGear_F/1
  EMS_RemindGear_S/1 -> EMS_RemindGearcv/1
  EMS_RemindGear_L/1 -> EMS_RemindGear_S/1
  EMS_RemindGear_Convert/1 -> EMS_RemindGear_L/1
  EMS_RemindGear_Sub/1(Out1) -> EMS_RemindGear_Convert/1
  EMS_RemindGear_sat/1 -> EMS_RemindGear_Out/1
  EMS_RemindGear_Ad/1 -> EMS_RemindGear_sat/1
  EMS_RemindGear_O/1 -> EMS_RemindGear_Ad/2
  EMS_RemindGear_F/1 -> EMS_RemindGear_Ad/1
  EPS_TorqueAssistModecv/1 -> EPS_TorqueAssistMode_F/1
  EPS_TorqueAssistMode_S/1 -> EPS_TorqueAssistModecv/1
  EPS_TorqueAssistMode_L/1 -> EPS_TorqueAssistMode_S/1
  EPS_TorqueAssistMode_Convert/1 -> EPS_TorqueAssistMode_L/1
  EPS_TorqueAssistMode_Sub/1(Out1) -> EPS_TorqueAssistMode_Convert/1
  Demux/1 -> TCU_FailureLamp_Sub/1(In1), EMS_RemindGear_Sub/1(In1), EPS_TorqueAssistMode_Sub/1(In1)
  EPS_TorqueAssistMode_sat/1 -> EPS_TorqueAssistMode_Out/1
  EPS_TorqueAssistMode_Ad/1 -> EPS_TorqueAssistMode_sat/1
  EPS_TorqueAssistMode_O/1 -> EPS_TorqueAssistMode_Ad/2
  EPS_TorqueAssistMode_F/1 -> EPS_TorqueAssistMode_Ad/1

== system VCU_CS75_9_30/长安CS75底盘程序，20ms一次/BSW_Input/CAN1_Rx/GW_567/ReceiveMessages/Subsystem/GW_2 ==
  input : Inport
  Demux : Demux  Outputs=8
  HU_Byroad_Ad : Sum
  HU_Byroad_Convert : DataTypeConversion  OutDataTypeStr=uint32
  HU_Byroad_F : Gain
  HU_Byroad_L : simulink/Logic and Bit Operations/Bitwise Operator  logicop=AND  UseBitMask=on  BitMask=192  BitMaskRealWorld=Stored Integer
  HU_Byroad_O : Constant  Value=0  OutDataTypeStr=single
  HU_Byroad_S : ArithShift  BitShiftNumber=6
  HU_Byroad_Sub : Subsystem
  HU_Byroad_sat : Saturate  UpperLimit=3  LowerLimit=0
  HU_Byroadcv : DataTypeConversion
  HU_EnterTunnelInfo_Ad : Sum
  HU_EnterTunnelInfo_Convert : DataTypeConversion  OutDataTypeStr=uint32
  HU_EnterTunnelInfo_F : Gain
  HU_EnterTunnelInfo_L : simulink/Logic and Bit Operations/Bitwise Operator  logicop=AND  UseBitMask=on  BitMask=12  BitMaskRealWorld=Stored Integer
  HU_EnterTunnelInfo_O : Constant  Value=0  OutDataTypeStr=single
  HU_EnterTunnelInfo_S : ArithShift  BitShiftNumber=2
  HU_EnterTunnelInfo_Sub : Subsystem
  HU_EnterTunnelInfo_sat : Saturate  UpperLimit=3  LowerLimit=0
  HU_EnterTunnelInfocv : DataTypeConversion
  HU_NavGuiganceStatus_Ad : Sum
  HU_NavGuiganceStatus_Convert : DataTypeConversion  OutDataTypeStr=uint32
  HU_NavGuiganceStatus_F : Gain
  HU_NavGuiganceStatus_L : simulink/Logic and Bit Operations/Bitwise Operator  logicop=AND  UseBitMask=on  BitMask=192  BitMaskRealWorld=Stored Integer
  HU_NavGuiganceStatus_O : Constant  Value=0  OutDataTypeStr=single
  HU_NavGuiganceStatus_S : ArithShift  BitShiftNumber=6
  HU_NavGuiganceStatus_Sub : Subsystem
  HU_NavGuiganceStatus_sat : Saturate  UpperLimit=3  LowerLimit=0
  HU_NavGuiganceStatuscv : DataTypeConversion
  HU_TunnelDistance_Ad : Sum
  HU_TunnelDistance_Convert : DataTypeConversion  OutDataTypeStr=uint32
  HU_TunnelDistance_F : Gain  Gain=10
  HU_TunnelDistance_L : simulink/Logic and Bit Operations/Bitwise Operator  logicop=AND  UseBitMask=on  BitMask=252  BitMaskRealWorld=Stored Integer
  HU_TunnelDistance_O : Constant  Value=0  OutDataTypeStr=single
  HU_TunnelDistance_S : ArithShift  BitShiftNumber=2
  HU_TunnelDistance_Sub : Subsystem
  HU_TunnelDistance_sat : Saturate  UpperLimit=600  LowerLimit=0
  HU_TunnelDistancecv : DataTypeConversion
  HU_TunnelLength_Ad : Sum
  HU_TunnelLength_Convert : DataTypeConversion  OutDataTypeStr=uint32
  HU_TunnelLength_F : Gain
  HU_TunnelLength_L : simulink/Logic and Bit Operations/Bitwise Operator  logicop=AND  UseBitMask=on  BitMask=63  BitMaskRealWorld=Stored Integer
  HU_TunnelLength_O : Constant  Value=0  OutDataTypeStr=single
  HU_TunnelLength_S : ArithShift
  HU_TunnelLength_Sub : Subsystem
  HU_TunnelLength_sat : Saturate  UpperLimit=63  LowerLimit=0
  HU_TunnelLengthcv : DataTypeConversion
  HU_EnterTunnelInfo_Out : Outport
  HU_TunnelDistance_Out : Outport  Port=2
  HU_TunnelLength_Out : Outport  Port=3
  HU_Byroad_Out : Outport  Port=4
  HU_NavGuiganceStatus_Out : Outport  Port=5
  wires:
  HU_EnterTunnelInfo_F/1 -> HU_EnterTunnelInfo_Ad/1
  HU_EnterTunnelInfo_O/1 -> HU_EnterTunnelInfo_Ad/2
  HU_EnterTunnelInfo_Ad/1 -> HU_EnterTunnelInfo_sat/1
  HU_EnterTunnelInfo_sat/1 -> HU_EnterTunnelInfo_Out/1
  Demux/1 -> HU_EnterTunnelInfo_Sub/1(In1)
  HU_EnterTunnelInfo_Sub/1(Out1) -> HU_EnterTunnelInfo_Convert/1
  HU_EnterTunnelInfo_Convert/1 -> HU_EnterTunnelInfo_L/1
  HU_EnterTunnelInfo_L/1 -> HU_EnterTunnelInfo_S/1
  HU_EnterTunnelInfo_S/1 -> HU_EnterTunnelInfocv/1
  HU_EnterTunnelInfocv/1 -> HU_EnterTunnelInfo_F/1
  HU_TunnelDistance_F/1 -> HU_TunnelDistance_Ad/1
  HU_TunnelDistance_O/1 -> HU_TunnelDistance_Ad/2
  HU_TunnelDistance_Ad/1 -> HU_TunnelDistance_sat/1
  HU_TunnelDistance_sat/1 -> HU_TunnelDistance_Out/1
  Demux/3 -> HU_TunnelDistance_Sub/1(In1)
  HU_TunnelDistance_Sub/1(Out1) -> HU_TunnelDistance_Convert/1
  HU_TunnelDistance_Convert/1 -> HU_TunnelDistance_L/1
  HU_TunnelDistance_L/1 -> HU_TunnelDistance_S/1
  HU_TunnelDistance_S/1 -> HU_TunnelDistancecv/1
  HU_TunnelDistancecv/1 -> HU_TunnelDistance_F/1
  HU_TunnelLength_F/1 -> HU_TunnelLength_Ad/1
  HU_TunnelLength_O/1 -> HU_TunnelLength_Ad/2
  HU_TunnelLength_Ad/1 -> HU_TunnelLength_sat/1
  HU_TunnelLength_sat/1 -> HU_TunnelLength_Out/1
  Demux/5 -> HU_TunnelLength_Sub/1(In1), HU_Byroad_Sub/1(In1)
  HU_TunnelLength_Sub/1(Out1) -> HU_TunnelLength_Convert/1
  HU_TunnelLength_Convert/1 -> HU_TunnelLength_L/1
  HU_TunnelLength_L/1 -> HU_TunnelLength_S/1
  HU_TunnelLength_S/1 -> HU_TunnelLengthcv/1
  HU_TunnelLengthcv/1 -> HU_TunnelLength_F/1
  HU_Byroad_F/1 -> HU_Byroad_Ad/1
  HU_Byroad_O/1 -> HU_Byroad_Ad/2
  HU_Byroad_Ad/1 -> HU_Byroad_sat/1
  HU_Byroad_sat/1 -> HU_Byroad_Out/1
  HU_Byroad_Sub/1(Out1) -> HU_Byroad_Convert/1
  HU_Byroad_Convert/1 -> HU_Byroad_L/1
  HU_Byroad_L/1 -> HU_Byroad_S/1
  HU_Byroad_S/1 -> HU_Byroadcv/1
  HU_Byroadcv/1 -> HU_Byroad_F/1
  HU_NavGuiganceStatus_F/1 -> HU_NavGuiganceStatus_Ad/1
  HU_NavGuiganceStatus_O/1 -> HU_NavGuiganceStatus_Ad/2
  HU_NavGuiganceStatus_Ad/1 -> HU_NavGuiganceStatus_sat/1
  HU_NavGuiganceStatus_sat/1 -> HU_NavGuiganceStatus_Out/1
  Demux/6 -> HU_NavGuiganceStatus_Sub/1(In1)
  HU_NavGuiganceStatus_Sub/1(Out1) -> HU_NavGuiganceStatus_Convert/1
  HU_NavGuiganceStatus_Convert/1 -> HU_NavGuiganceStatus_L/1
  HU_NavGuiganceStatus_L/1 -> HU_NavGuiganceStatus_S/1
  HU_NavGuiganceStatus_S/1 -> HU_NavGuiganceStatuscv/1
  HU_NavGuiganceStatuscv/1 -> HU_NavGuiganceStatus_F/1
  input/1 -> Demux/1

== system VCU_CS75_9_30/长安CS75底盘程序，20ms一次/BSW_Input/CAN1_Rx/HU_GPS_500/ReceiveMessages/Subsystem/HU_GPS_1 ==
  input : Inport
  Demux : Demux  Outputs=8
  GPSCurrentLocationValid_Ad : Sum
  GPSCurrentLocationValid_Convert : DataTypeConversion  OutDataTypeStr=uint32
  GPSCurrentLocationValid_F : Gain
  GPSCurrentLocationValid_L : simulink/Logic and Bit Operations/Bitwise Operator  logicop=AND  UseBitMask=on  BitMask=128  BitMaskRealWorld=Stored Integer
  GPSCurrentLocationValid_O : Constant  Value=0  OutDataTypeStr=single
  GPSCurrentLocationValid_S : ArithShift  BitShiftNumber=7
  GPSCurrentLocationValid_Sub : Subsystem
  GPSCurrentLocationValid_sat : Saturate  UpperLimit=0  LowerLimit=0
  GPSCurrentLocationValidcv : DataTypeConversion
  GPSCurrentLocationValid_Out : Outport
  wires:
  input/1 -> Demux/1
  GPSCurrentLocationValidcv/1 -> GPSCurrentLocationValid_F/1
  GPSCurrentLocationValid_S/1 -> GPSCurrentLocationValidcv/1
  GPSCurrentLocationValid_L/1 -> GPSCurrentLocationValid_S/1
  GPSCurrentLocationValid_Convert/1 -> GPSCurrentLocationValid_L/1
  GPSCurrentLocationValid_Sub/1(Out1) -> GPSCurrentLocationValid_Convert/1
  Demux/1 -> GPSCurrentLocationValid_Sub/1(In1)
  GPSCurrentLocationValid_sat/1 -> GPSCurrentLocationValid_Out/1
  GPSCurrentLocationValid_Ad/1 -> GPSCurrentLocationValid_sat/1
  GPSCurrentLocationValid_O/1 -> GPSCurrentLocationValid_Ad/2
  GPSCurrentLocationValid_F/1 -> GPSCurrentLocationValid_Ad/1

== system VCU_CS75_9_30/长安CS75底盘程序，20ms一次/BSW_Input/CAN1_Rx/LAS_36E/ReceiveMessages/Subsystem/LAS_36E2 ==
  input : Inport
  Demux : Demux  Outputs=8
  LAS_CheckSum_id36E_Ad : Sum
  LAS_CheckSum_id36E_Convert : DataTypeConversion  OutDataTypeStr=uint32
  LAS_CheckSum_id36E_F : Gain
  LAS_CheckSum_id36E_L : simulink/Logic and Bit Operations/Bitwise Operator  logicop=AND  UseBitMask=on  BitMask=255  BitMaskRealWorld=Stored Integer
  LAS_CheckSum_id36E_O : Constant  Value=0  OutDataTypeStr=single
  LAS_CheckSum_id36E_S : ArithShift
  LAS_CheckSum_id36E_Sub : Subsystem
  LAS_CheckSum_id36E_sat : Saturate  UpperLimit=255  LowerLimit=0
  LAS_CheckSum_id36Ecv : DataTypeConversion
  LAS_LaneEquationC1_Ad : Sum
  LAS_LaneEquationC1_Convert : DataTypeConversion  OutDataTypeStr=uint32
  LAS_LaneEquationC1_F : Gain  Gain=0.00048828125
  LAS_LaneEquationC1_L : simulink/Logic and Bit Operations/Bitwise Operator  logicop=AND  UseBitMask=on  BitMask=262080  BitMaskRealWorld=Stored Integer
  LAS_LaneEquationC1_O : Constant  Value=-1  OutDataTypeStr=single
  LAS_LaneEquationC1_S : ArithShift  BitShiftNumber=6
  LAS_LaneEquationC1_Sub : Subsystem
  LAS_LaneEquationC1_sat : Saturate  UpperLimit=0.9990234375  LowerLimit=-1
  LAS_LaneEquationC1cv : DataTypeConversion
  LAS_LaneEquationC1input2_Ad : Sum
  LAS_LaneEquationC1input2_C : Constant  Value=65536
  LAS_LaneEquationC1input2_P : Product
  LAS_LaneEquationC1input3_Ad : Sum
  LAS_LaneEquationC1input3_C : Constant  Value=256
  LAS_LaneEquationC1input3_P : Product
  LAS_LaneEquationC3_Ad : Sum
  LAS_LaneEquationC3_Convert : DataTypeConversion  OutDataTypeStr=uint32
  LAS_LaneEquationC3_F : Gain  Gain=4.76837158203125
  LAS_LaneEquationC3_L : simulink/Logic and Bit Operations/Bitwise Operator  logicop=AND  UseBitMask=on  BitMask=262080  BitMaskRealWorld=Stored Integer
  LAS_LaneEquationC3_O : Constant  Value=-0.000976085662841796  OutDataTypeStr=single
  LAS_LaneEquationC3_S : ArithShift  BitShiftNumber=6
  LAS_LaneEquationC3_Sub : Subsystem
  LAS_LaneEquationC3_sat : Saturate  UpperLimit=0.000976085662841796  LowerLimit=-0.000976085662841796
  LAS_LaneEquationC3cv : DataTypeConversion
  LAS_LaneEquationC3input5_Ad : Sum
  LAS_LaneEquationC3input5_C : Constant  Value=65536
  LAS_LaneEquationC3input5_P : Product
  LAS_LaneEquationC3input6_Ad : Sum
  LAS_LaneEquationC3input6_C : Constant  Value=256
  LAS_LaneEquationC3input6_P : Product
  LAS_LaneEquationStatus_Ad : Sum
  LAS_LaneEquationStatus_Convert : DataTypeConversion  OutDataTypeStr=uint32
  LAS_LaneEquationStatus_F : Gain
  LAS_LaneEquationStatus_L : simulink/Logic and Bit Operations/Bitwise Operator  logicop=AND  UseBitMask=on  BitMask=48  BitMaskRealWorld=Stored Integer
  LAS_LaneEquationStatus_O : Constant  Value=0  OutDataTypeStr=single
  LAS_LaneEquationStatus_S : ArithShift  BitShiftNumber=4
  LAS_LaneEquationStatus_Sub : Subsystem
  LAS_LaneEquationStatus_sat : Saturate  UpperLimit=3  LowerLimit=0
  LAS_LaneEquationStatuscv : DataTypeConversion
  LAS_RoadCurvatureFar_Ad : Sum
  LAS_RoadCurvatureFar_Convert : DataTypeConversion  OutDataTypeStr=uint32
  LAS_RoadCurvatureFar_F : Gain  Gain=0.0005
  LAS_RoadCurvatureFar_L : simulink/Logic and Bit Operations/Bitwise Operator  logicop=AND  UseBitMask=on  BitMask=508  BitMaskRealWorld=Stored Integer
  LAS_RoadCurvatureFar_O : Constant  Value=-0.03  OutDataTypeStr=single
  LAS_RoadCurvatureFar_S : ArithShift  BitShiftNumber=2
  LAS_RoadCurvatureFar_Sub : Subsystem
  LAS_RoadCurvatureFar_sat : Saturate  UpperLimit=0.03  LowerLimit=-0.03
  LAS_RoadCurvatureFarcv : DataTypeConversion
  LAS_RoadCurvatureFarinput1_Ad : Sum
  LAS_RoadCurvatureFarinput1_C : Constant  Value=256
  LAS_RoadCurvatureFarinput1_P : Product
  LAS_RoadCurvatureNear_Ad : Sum
  LAS_RoadCurvatureNear_Convert : DataTypeConversion  OutDataTypeStr=uint32
  LAS_RoadCurvatureNear_F : Gain  Gain=0.0005
  LAS_RoadCurvatureNear_L : simulink/Logic and Bit Operations/Bitwise Operator  logicop=AND  UseBitMask=on  BitMask=254  BitMaskRealWorld=Stored Integer
  LAS_RoadCurvatureNear_O : Constant  Value=-0.03  OutDataTypeStr=single
  LAS_RoadCurvatureNear_S : ArithShift  BitShiftNumber=1
  LAS_RoadCurvatureNear_Sub : Subsystem
  LAS_RoadCurvatureNear_sat : Saturate  UpperLimit=0.03  LowerLimit=-0.03
  LAS_RoadCurvatureNearcv : DataTypeConversion
  LAS_RollingCounter_id36E_Ad : Sum
  LAS_RollingCounter_id36E_Convert : DataTypeConversion  OutDataTypeStr=uint32
  LAS_RollingCounter_id36E_F : Gain
  LAS_RollingCounter_id36E_L : simulink/Logic and Bit Operations/Bitwise Operator  logicop=AND  UseBitMask=on  BitMask=15  BitMaskRealWorld=Stored Integer
  LAS_RollingCounter_id36E_O : Constant  Value=0  OutDataTypeStr=single
  LAS_RollingCounter_id36E_S : ArithShift
  LAS_RollingCounter_id36E_Sub : Subsystem
  LAS_RollingCounter_id36E_sat : Saturate  UpperLimit=15  LowerLimit=0
  LAS_RollingCounter_id36Ecv : DataTypeConversion
  LAS_RoadCurvatureFar_Out : Outport
  LAS_RoadCurvatureNear_Out : Outport  Port=2
  LAS_LaneEquationC1_Out : Outport  Port=3
  LAS_LaneEquationC3_Out : Outport  Port=4
  LAS_RollingCounter_id36E_Out : Outport  Port=5
  LAS_LaneEquationStatus_Out : Outport  Port=6
  LAS_CheckSum_id36E_Out : Outport  Port=7
  wires:
  LAS_RoadCurvatureFar_F/1 -> LAS_RoadCurvatureFar_Ad/1
  LAS_RoadCurvatureFar_O/1 -> LAS_RoadCurvatureFar_Ad/2
  LAS_RoadCurvatureFar_Ad/1 -> LAS_RoadCurvatureFar_sat/1
  LAS_RoadCurvatureFar_sat/1 -> LAS_RoadCurvatureFar_Out/1
  Demux/1 -> LAS_RoadCurvatureFarinput1_P/1, LAS_RoadCurvatureNear_Sub/1(In1)
  LAS_RoadCurvatureFarinput1_C/1 -> LAS_RoadCurvatureFarinput1_P/2
  LAS_RoadCurvatureFarinput1_P/1 -> LAS_RoadCurvatureFarinput1_Ad/1
  Demux/2 -> LAS_RoadCurvatureFarinput1_Ad/2, LAS_LaneEquationC1input2_P/1
  LAS_RoadCurvatureFarinput1_Ad/1 -> LAS_RoadCurvatureFar_Sub/1(In1)
  LAS_RoadCurvatureFar_Sub/1(Out1) -> LAS_RoadCurvatureFar_Convert/1
  LAS_RoadCurvatureFar_Convert/1 -> LAS_RoadCurvatureFar_L/1
  LAS_RoadCurvatureFar_L/1 -> LAS_RoadCurvatureFar_S/1
  LAS_RoadCurvatureFar_S/1 -> LAS_RoadCurvatureFarcv/1
  LAS_RoadCurvatureFarcv/1 -> LAS_RoadCurvatureFar_F/1
  LAS_RoadCurvatureNear_F/1 -> LAS_RoadCurvatureNear_Ad/1
  LAS_RoadCurvatureNear_O/1 -> LAS_RoadCurvatureNear_Ad/2
  LAS_RoadCurvatureNear_Ad/1 -> LAS_RoadCurvatureNear_sat/1
  LAS_RoadCurvatureNear_sat/1 -> LAS_RoadCurvatureNear_Out/1
  LAS_RoadCurvatureNear_Sub/1(Out1) -> LAS_RoadCurvatureNear_Convert/1
  LAS_RoadCurvatureNear_Convert/1 -> LAS_RoadCurvatureNear_L/1
  LAS_RoadCurvatureNear_L/1 -> LAS_RoadCurvatureNear_S/1
  LAS_RoadCurvatureNear_S/1 -> LAS_RoadCurvatureNearcv/1
  LAS_RoadCurvatureNearcv/1 -> LAS_RoadCurvatureNear_F/1
  LAS_LaneEquationC1_F/1 -> LAS_LaneEquationC1_Ad/1
  LAS_LaneEquationC1_O/1 -> LAS_LaneEquationC1_Ad/2
  LAS_LaneEquationC1_Ad/1 -> LAS_LaneEquationC1_sat/1
  LAS_LaneEquationC1_sat/1 -> LAS_LaneEquationC1_Out/1
  LAS_LaneEquationC1input2_C/1 -> LAS_LaneEquationC1input2_P/2
  LAS_LaneEquationC1input2_P/1 -> LAS_LaneEquationC1input2_Ad/1
  Demux/4 -> LAS_LaneEquationC1input2_Ad/2
  Demux/3 -> LAS_LaneEquationC1input3_P/1
  LAS_LaneEquationC1input3_C/1 -> LAS_LaneEquationC1input3_P/2
  LAS_LaneEquationC1input3_P/1 -> LAS_LaneEquationC1input3_Ad/1
  LAS_LaneEquationC1input2_Ad/1 -> LAS_LaneEquationC1input3_Ad/2
  LAS_LaneEquationC1input3_Ad/1 -> LAS_LaneEquationC1_Sub/1(In1)
  LAS_LaneEquationC1_Sub/1(Out1) -> LAS_LaneEquationC1_Convert/1
  LAS_LaneEquationC1_Convert/1 -> LAS_LaneEquationC1_L/1
  LAS_LaneEquationC1_L/1 -> LAS_LaneEquationC1_S/1
  LAS_LaneEquationC1_S/1 -> LAS_LaneEquationC1cv/1
  LAS_LaneEquationC1cv/1 -> LAS_LaneEquationC1_F/1
  LAS_LaneEquationC3_F/1 -> LAS_LaneEquationC3_Ad/1
  LAS_LaneEquationC3_O/1 -> LAS_LaneEquationC3_Ad/2
  LAS_LaneEquationC3_Ad/1 -> LAS_LaneEquationC3_sat/1
  LAS_LaneEquationC3_sat/1 -> LAS_LaneEquationC3_Out/1
  Demux/5 -> LAS_LaneEquationC3input5_P/1
  LAS_LaneEquationC3input5_C/1 -> LAS_LaneEquationC3input5_P/2
  LAS_LaneEquationC3input5_P/1 -> LAS_LaneEquationC3input5_Ad/1
  Demux/7 -> LAS_LaneEquationC3input5_Ad/2, LAS_RollingCounter_id36E_Sub/1(In1), LAS_LaneEquationStatus_Sub/1(In1)
  Demux/6 -> LAS_LaneEquationC3input6_P/1
  LAS_LaneEquationC3input6_C/1 -> LAS_LaneEquationC3input6_P/2
  LAS_LaneEquationC3input6_P/1 -> LAS_LaneEquationC3input6_Ad/1
  LAS_LaneEquationC3input5_Ad/1 -> LAS_LaneEquationC3input6_Ad/2
  LAS_LaneEquationC3input6_Ad/1 -> LAS_LaneEquationC3_Sub/1(In1)
  LAS_LaneEquationC3_Sub/1(Out1) -> LAS_LaneEquationC3_Convert/1
  LAS_LaneEquationC3_Convert/1 -> LAS_LaneEquationC3_L/1
  LAS_LaneEquationC3_L/1 -> LAS_LaneEquationC3_S/1
  LAS_LaneEquationC3_S/1 -> LAS_LaneEquationC3cv/1
  LAS_LaneEquationC3cv/1 -> LAS_LaneEquationC3_F/1
  LAS_RollingCounter_id36E_F/1 -> LAS_RollingCounter_id36E_Ad/1
  LAS_RollingCounter_id36E_O/1 -> LAS_RollingCounter_id36E_Ad/2
  LAS_RollingCounter_id36E_Ad/1 -> LAS_RollingCounter_id36E_sat/1
  LAS_RollingCounter_id36E_sat/1 -> LAS_RollingCounter_id36E_Out/1
  LAS_RollingCounter_id36E_Sub/1(Out1) -> LAS_RollingCounter_id36E_Convert/1
  LAS_RollingCounter_id36E_Convert/1 -> LAS_RollingCounter_id36E_L/1
  LAS_RollingCounter_id36E_L/1 -> LAS_RollingCounter_id36E_S/1
  LAS_RollingCounter_id36E_S/1 -> LAS_RollingCounter_id36Ecv/1
  LAS_RollingCounter_id36Ecv/1 -> LAS_RollingCounter_id36E_F/1
  LAS_LaneEquationStatus_F/1 -> LAS_LaneEquationStatus_Ad/1
  LAS_LaneEquationStatus_O/1 -> LAS_LaneEquationStatus_Ad/2
  LAS_LaneEquationStatus_Ad/1 -> LAS_LaneEquationStatus_sat/1
  LAS_LaneEquationStatus_sat/1 -> LAS_LaneEquationStatus_Out/1
  LAS_LaneEquationStatus_Sub/1(Out1) -> LAS_LaneEquationStatus_Convert/1
  LAS_LaneEquationStatus_Convert/1 -> LAS_LaneEquationStatus_L/1
  LAS_LaneEquationStatus_L/1 -> LAS_LaneEquationStatus_S/1
  LAS_LaneEquationStatus_S/1 -> LAS_LaneEquationStatuscv/1
  LAS_LaneEquationStatuscv/1 -> LAS_LaneEquationStatus_F/1
  LAS_CheckSum_id36E_F/1 -> LAS_CheckSum_id36E_Ad/1
  LAS_CheckSum_id36E_O/1 -> LAS_CheckSum_id36E_Ad/2
  LAS_CheckSum_id36E_Ad/1 -> LAS_CheckSum_id36E_sat/1
  LAS_CheckSum_id36E_sat/1 -> LAS_CheckSum_id36E_Out/1
  Demux/8 -> LAS_CheckSum_id36E_Sub/1(In1)
  LAS_CheckSum_id36E_Sub/1(Out1) -> LAS_CheckSum_id36E_Convert/1
  LAS_CheckSum_id36E_Convert/1 -> LAS_CheckSum_id36E_L/1
  LAS_CheckSum_id36E_L/1 -> LAS_CheckSum_id36E_S/1
  LAS_CheckSum_id36E_S/1 -> LAS_CheckSum_id36Ecv/1
  LAS_CheckSum_id36Ecv/1 -> LAS_CheckSum_id36E_F/1
  input/1 -> Demux/1
